simulink model "Traffic_controller_MILTest"  (R2024b)
settings: Solver=FixedStepAuto  StartTime=0.0  StopTime=1  RelTol=1e-3  EnableMultiTasking=on
libraries: SignalEditorBlockLib x1
settings Model: ExtModeTrigDuration=2  Creator=Sagar  LastModifiedBy=Sagar
settings SolverCC: AutoInsertRateTranBlk=on
settings OptimizationCC: EnhancedBackFolding=on  PassReuseOutputArgsAs=Individual arguments  ZeroExternalMemoryAtStartup=off  ZeroInternalMemoryAtStartup=off  MaxStackSize=64  OptimizeBlockOrder=speed  DifferentSizesBufferReuse=on  OptimizationCustomize=off  EfficientTunableParamExpr=on
settings DebuggingCC: SignalInfNanChecking=error  CheckMatrixSingularityMsg=error  IntegerOverflowMsg=error  ParameterTunabilityLossMsg=error  UnderSpecifiedDataTypeMsg=error  SignalLabelMismatchMsg=error  UnconnectedInputMsg=error  UnconnectedOutputMsg=error  UnconnectedLineMsg=error  UniqueDataStoreMsg=error  IntegerSaturationMsg=error
settings HardwareCC: ProdBitPerInt=16  ProdBitPerPointer=16  ProdBitPerSizeT=16  ProdBitPerPtrDiffT=16  ProdLargestAtomicFloat=None  ProdWordSize=8  ProdHWDeviceType=Atmel->AVR
settings SFSimCC: MATLABDynamicMemAlloc=off
settings RTWCC: Description=Embedded Coder  SystemTargetFile=ert.tlc  HardwareBoard=Arduino Mega 2560  TemplateMakefile=ert_default_tmf  Toolchain=Arduino AVR  BuildConfiguration=Faster Runs
settings CodeAppCC: ForceParamTrailComments=on  IgnoreCustomStorageClasses=off  OperatorAnnotations=on  SimulinkDataObjDesc=on  SFDataObjDesc=on  InsertBlockDesc=on
settings ERTTargetCC: SupportContinuousTime=on  SupportVariableSizeSignals=on  ExtModeTransport=3  ExtModeStaticAlloc=on  ExtModeAutomaticAllocSize=off  ExtModeStaticAllocSize=2048  ExtModeMexFile=ext_xcp  ExtModeIntrfLevel=Level2 - Open  InlinedParameterPlacement=Hierarchical
settings ConfigComp: CovMetricSettings=dcmwe

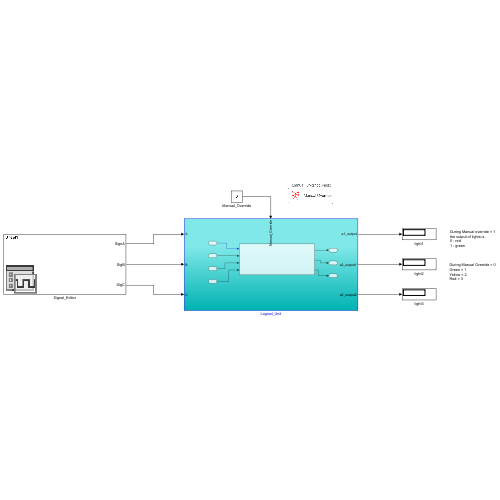
[thumbnail: Simulink's stored preview of the top-level diagram]
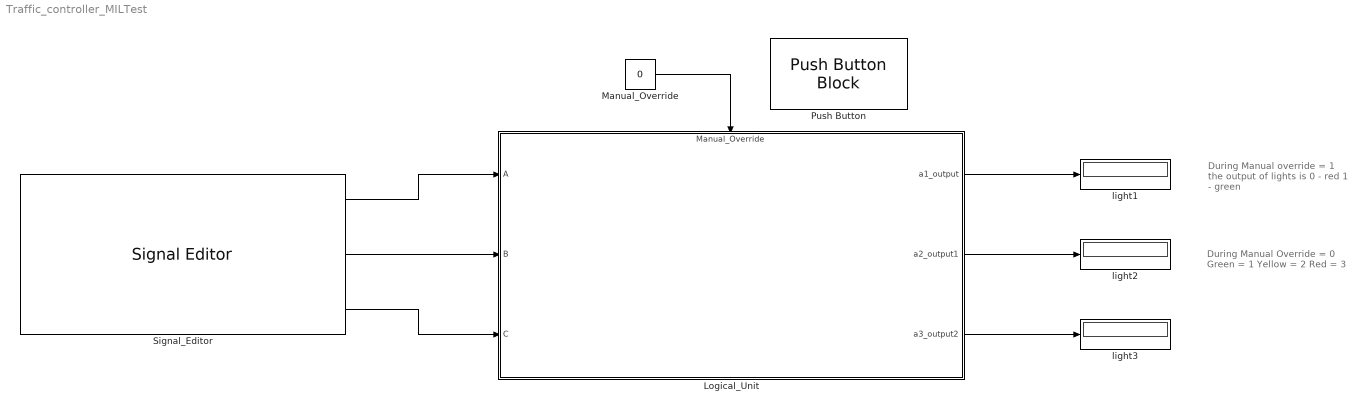
== system Traffic_controller_MILTest ==
  note: During Manual Override = 0
      | Green = 1
      | Yellow = 2
      | Red = 3
  note: During Manual override = 1
      | the output of lights is
      | 0 - red
      | 1 - green
  Logical_Unit : Subsystem
      settings: PortSchema="{\"entries\":[{\"content\":{\"sides\":[{\"content\":{\"connectorIds\":[\"In1\",\"In2\",\"In3\"]},\"type\":\"ConnectorPlacement.EquallySpacedRectSide\",\"uuid\":\"8855ce6d-d1ff-4d7f-a3df-67bdf88ab5f5\"},{\"content\":{\"connectorIds\":[\"Out1\",\"Out2\",\"Out3\"],\"side\":\"RIGHT\"},\"type\":\"ConnectorPlacement.EquallySpacedRectSide\",\"uuid\":\"52f56ae2-25c7-4c8f-a76f-4a07a3778792\"},{\"content\":{\"connectorIds\":[\"In4\"],\"side\":\"TOP\"},\"type\":\"ConnectorPlacement.EquallySpacedRectSide\",\"uuid\":\"7fe2cf04-5da7-44c6-9157-4fd5825aeae5\"}]},\"type\":\"ConnectorPlacement.EquallySpacedConnector\",\"uuid\":\"d49c1084-20b5-4dd5-a2b8-171e20c1de77\"}],\"packageUris\":[\"http://schema.mathworks.com/mf0/Connector/R2020b\"],\"version\":\"1.0\"}"
  Manual_Override : Constant  Value=0
  Push Button : PushButtonBlock  LabelPosition=Top  ButtonText=Manual Override  ButtonType=Latch  Icon=NetworkTransmission  IconColor=On  OffValue=0.000000
  Signal_Editor : SignalEditorBlockLib/Signal Editor  FileName=Test.mat  ActiveScenario=Sheet1  ActiveSignal=SignA  IsBus=off  OutputBusObjectStr=Bus: BusObject  SampleTime=0  Interpolate=off  ZeroCross=off  OutputAfterFinalValue=Setting to zero  Unit=inherit  PreserveSignalName=on  ApplySigPropsToAllScenarios=on  ApplySigPropsToAllSignals=off
  light1 : Display
  light2 : Display
  light3 : Display
  wires:
  Logical_Unit/1(a1_output) -> light1/1
  Manual_Override/1 -> Logical_Unit/4(Manual_Override)
  Logical_Unit/2(a2_output1) -> light2/1
  Logical_Unit/3(a3_output2) -> light3/1
  Signal_Editor/3 -> Logical_Unit/3(C)
  Signal_Editor/2 -> Logical_Unit/2(B)
  Signal_Editor/1 -> Logical_Unit/1(A)

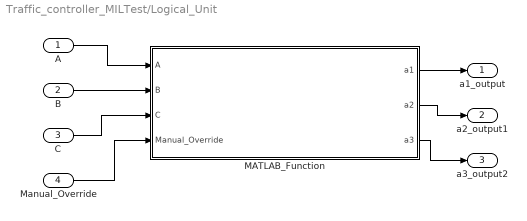
== system Traffic_controller_MILTest/Logical_Unit ==
  A : Inport
  B : Inport  Port=2
  C : Inport  Port=3
  Manual_Override : Inport  Port=4
  MATLAB_Function : MATLAB Function  TreatAsAtomicUnit=on
  a1_output : Outport
  a2_output1 : Outport  Port=2
  a3_output2 : Outport  Port=3
  wires:
  C/1 -> MATLAB_Function/3(C)
  B/1 -> MATLAB_Function/2(B)
  A/1 -> MATLAB_Function/1(A)
  MATLAB_Function/1(a1) -> a1_output/1
  Manual_Override/1 -> MATLAB_Function/4(Manual_Override)
  MATLAB_Function/3(a3) -> a3_output2/1
  MATLAB_Function/2(a2) -> a2_output1/1

== matlab function Traffic_controller_MILTest/Logical_Unit/MATLAB_Function ==
  data: A input; a1 output; B input; C input; Manual_Override input; a2 output; a3 output
function [a1, a2, a3] = fcn(A, B, C, Manual_Override)
    % Initialize outputs
    a1 = 0;
    a2 = 0;
    a3 = 0;

    % Manual Override Mode
    if Manual_Override == 1
        if A == 99
            a1 = 1;
            a2 = 0;
            a3 = 0;
        elseif B == 99
            a1 = 0;
            a2 = 1;
            a3 = 0;
        elseif C == 99
            a1 = 0;
            a2 = 0;
            a3 = 1;
        end
    else
        % Automatic Mode (Traffic Light Logic)
        if A > B && B > C
            disp("A = green");
            disp("B = yellow");
            disp("C = red");
            a1 = 1; % Green
            a2 = 2; % Yellow
            a3 = 3; % Red
        elseif B > C && C > A
            disp("A = red");
            disp("B = green");
            disp("C = yellow");
            a1 = 3; % Red
            a2 = 1; % Green
            a3 = 2; % Yellow
        elseif C > A && A > B
            disp("A = yellow");
            disp("B = red");
            disp("C = green");
            a1 = 2; % Yellow
            a2 = 3; % Red
            a3 = 1; % Green
        else
            disp("Invalid input or equal values.");
        end
    end
end
